simulink model "buck_converter_VMC"  (R2021a)
settings: Solver=VariableStepAuto  StartTime=0.0  StopTime=t_sim  RelTol=1e-3
values from neighbouring files (symbols this model uses):
  C = 600e-6    (= 0.0006)    [boost_parameters.m]    (also in buck_parameters.m = 0.0002)
  D = (Vref-Vin)/Vref    (= 0.5)    [boost_parameters.m]    (also in buck_parameters.m = 0.1; small_signal_model.m = 0.1)
  iL_0 = 0    [boost_parameters.m]    (also in buck_parameters.m)
  L = 50e-6    (= 5e-05)    [boost_parameters.m]    (also in buck_parameters.m = 5e-07)
  R = 1    [boost_parameters.m]    (also in buck_parameters.m; small_signal_model.m = 10; soft_start.m; soft_start_feedforward_backward.m)
  r_1 = 5e-3    (= 0.005)    [boost_parameters.m]    (also in buck_parameters.m)
  r_2 = 5e-3    (= 0.005)    [boost_parameters.m]    (also in buck_parameters.m)
  r_C = 3e-3    (= 0.003)    [boost_parameters.m]    (also in buck_parameters.m)
  r_L = 5e-3    (= 0.005)    [boost_parameters.m]    (also in buck_parameters.m)
  T = 2e-6    (= 2e-06)    [boost_parameters.m]    (also in buck_parameters.m)
  V_max = 10    [boost_parameters.m]
  V_min = 0    [boost_parameters.m]
  vC_0 = 0    [boost_parameters.m]    (also in buck_parameters.m)
  Vin = 12    [boost_parameters.m]    (also in buck_parameters.m; small_signal_model.m)
  Vref = 24    [boost_parameters.m]    (also in buck_parameters.m = 1.2; small_signal_model.m = 1.2)
undefined symbols (not defined in the file or in its folder): Kp
libraries: simulink x1, simulink_extras x1
settings Model: Creator=Hari Prasad Adhikari  LastModifiedBy=Hari Prasad Adhikari

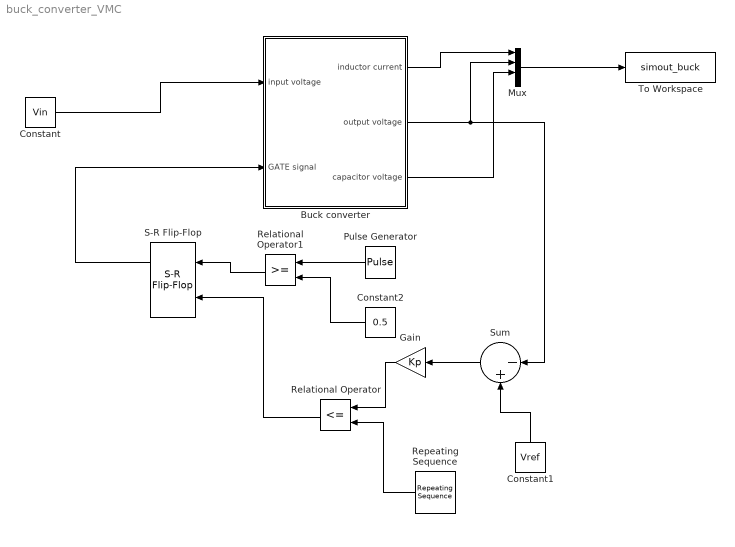
== system buck_converter_VMC ==
  Buck converter : Subsystem
  Constant : Constant  Value=Vin
  Constant1 : Constant  Value=Vref
  Constant2 : Constant  Value=0.5
  Gain : Gain  Gain=Kp
  Mux : Mux
  Pulse Generator : DiscretePulseGenerator  PulseType=Time based  Period=T  PulseWidth=D*100
  Relational Operator : RelationalOperator  Operator=<=  OutDataTypeStr=boolean  RndMeth=Simplest
  Relational Operator1 : RelationalOperator  OutDataTypeStr=boolean  RndMeth=Simplest
  Repeating Sequence : simulink/Sources/Repeating Sequence  rep_seq_t=[0 T]  rep_seq_y=[V_min V_max]
  S-R Flip-Flop : simulink_extras/Flip Flops/S-R Flip-Flop  initial_condition=0
  Sum : Sum  Inputs=|-+
  To Workspace : ToWorkspace  VariableName=simout_buck  SaveFormat=Timeseries  SampleTime=-1
  wires:
  Constant/1 -> Buck converter/1(input voltage)
  Buck converter/1(inductor current) -> Mux/1
  Buck converter/2(output voltage) -> Sum/1, Mux/2
  Buck converter/3(capacitor voltage) -> Mux/3
  Mux/1 -> To Workspace/1
  Sum/1 -> Gain/1
  Repeating Sequence/1 -> Relational Operator/2
  Pulse Generator/1 -> Relational Operator1/1
  Constant2/1 -> Relational Operator1/2
  Relational Operator1/1 -> S-R Flip-Flop/1
  Relational Operator/1 -> S-R Flip-Flop/2
  S-R Flip-Flop/1 -> Buck converter/2(GATE signal)
  Constant1/1 -> Sum/2
  Gain/1 -> Relational Operator/1

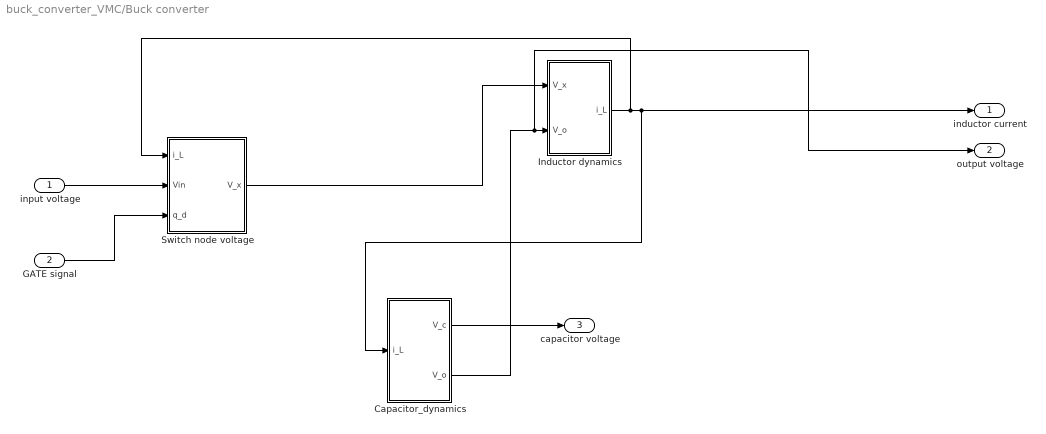
== system buck_converter_VMC/Buck converter ==
  input voltage : Inport
  GATE signal : Inport  Port=2
  Capacitor_dynamics : Subsystem
  Inductor dynamics : Subsystem
  Switch node voltage : Subsystem
  inductor current : Outport
  output voltage : Outport  Port=2
  capacitor voltage : Outport  Port=3
  wires:
  Capacitor_dynamics/1(V_c) -> capacitor voltage/1
  Inductor dynamics/1(i_L) -> inductor current/1, Capacitor_dynamics/1(i_L), Switch node voltage/1(i_L)
  Capacitor_dynamics/2(V_o) -> output voltage/1, Inductor dynamics/2(V_o)
  Switch node voltage/1(V_x) -> Inductor dynamics/1(V_x)
  GATE signal/1 -> Switch node voltage/3(q_d)
  input voltage/1 -> Switch node voltage/2(Vin)

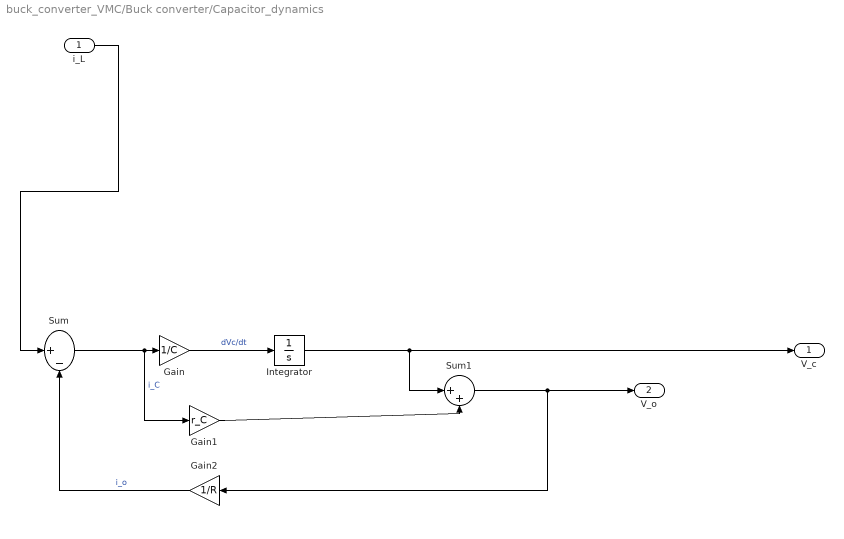
== system buck_converter_VMC/Buck converter/Capacitor_dynamics ==
  i_L : Inport
  Gain : Gain  Gain=1/C
  Gain1 : Gain  Gain=r_C
  Gain2 : Gain  Gain=1/R
  Integrator : Integrator  InitialCondition=vC_0
  Sum : Sum  Inputs=|+-
  Sum1 : Sum  Inputs=|++
  V_c : Outport
  V_o : Outport  Port=2
  wires:
  Integrator/1 -> V_c/1, Sum1/1
  Sum1/1 -> V_o/1, Gain2/1
  Gain1/1 -> Sum1/2
  Sum/1 -> Gain1/1, Gain/1  "i_C"
  Gain2/1 -> Sum/2  "i_o"
  Gain/1 -> Integrator/1  "dVc/dt"
  i_L/1 -> Sum/1

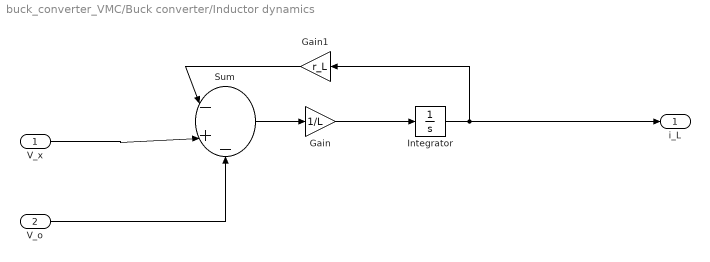
== system buck_converter_VMC/Buck converter/Inductor dynamics ==
  V_x : Inport
  V_o : Inport  Port=2
  Gain : Gain  Gain=1/L
  Gain1 : Gain  Gain=r_L
  Integrator : Integrator  InitialCondition=iL_0
  Sum : Sum  Inputs=|-+-
  i_L : Outport
  wires:
  Integrator/1 -> i_L/1, Gain1/1
  Gain/1 -> Integrator/1
  V_o/1 -> Sum/3
  Sum/1 -> Gain/1
  Gain1/1 -> Sum/1
  V_x/1 -> Sum/2

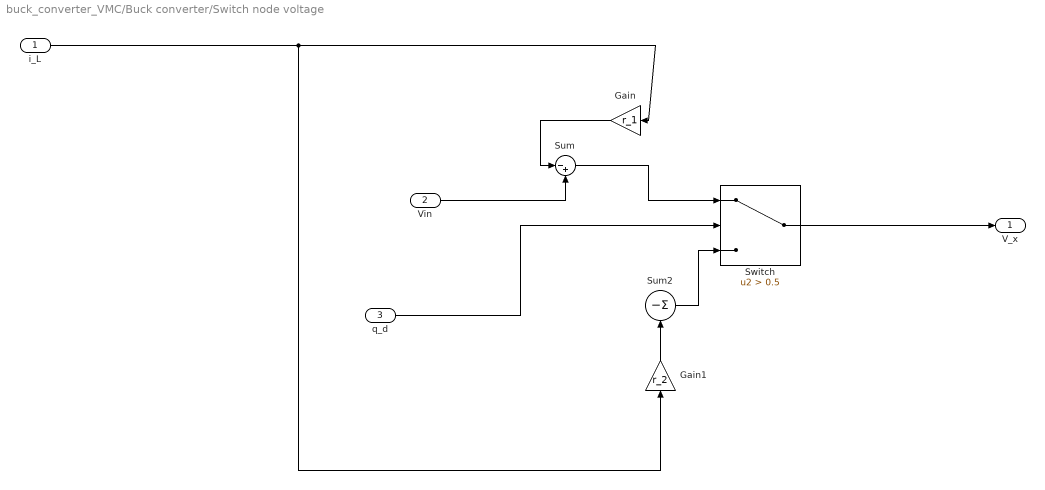
== system buck_converter_VMC/Buck converter/Switch node voltage ==
  i_L : Inport
  Vin : Inport  Port=2
  q_d : Inport  Port=3
  Gain : Gain  Gain=r_1
  Gain1 : Gain  Gain=r_2
  Sum : Sum  Inputs=|-+
  Sum2 : Sum  Inputs=|-
  Switch : Switch  Criteria=u2 > Threshold  Threshold=0.5
  V_x : Outport
  wires:
  Gain/1 -> Sum/1
  Gain1/1 -> Sum2/1
  i_L/1 -> Gain1/1, Gain/1
  Switch/1 -> V_x/1
  Sum/1 -> Switch/1
  q_d/1 -> Switch/2
  Sum2/1 -> Switch/3
  Vin/1 -> Sum/2
